simulink model "projeto_final"  (Simulink 6.3)
settings: Solver=ode3  StartTime=0  StopTime=5e-3  FixedStep=1e-7  RelTol=1e-3
undefined symbols (not defined in the file or in its folder): Fs, get
libraries: dsparch4 x1, commsynccomp2 x1, dspsnks4 x1
settings Model: LastModifiedBy=marco

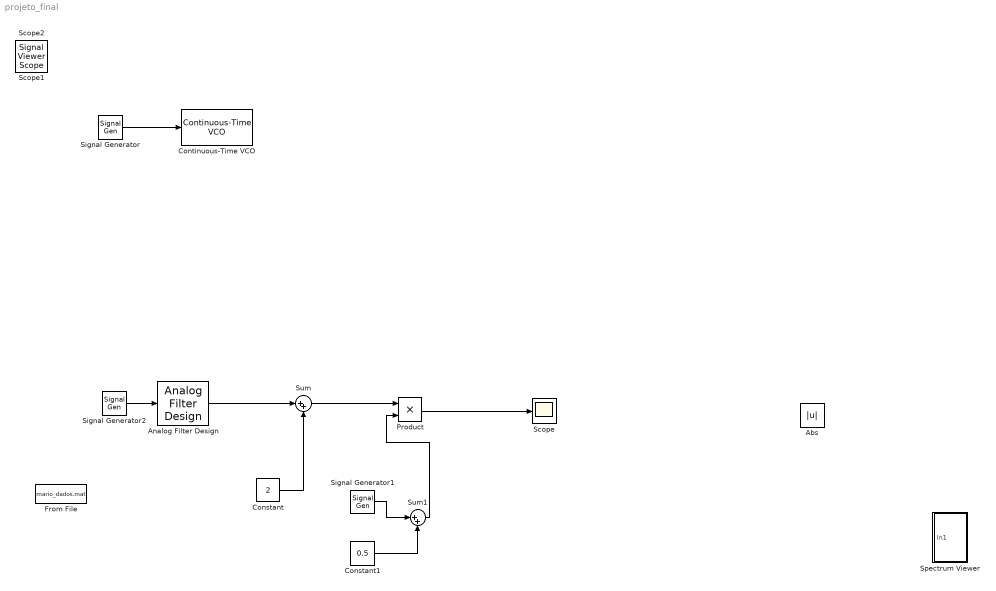
== system projeto_final ==
  Abs : Abs
  Analog Filter Design : dsparch4/Analog Filter Design  method=Butterworth  filttype=Lowpass  N=10  Wlo=2*pi*5e3  Whi=80  Rp=2  Rs=40
  Constant : Constant  Value=2
  Constant1 : Constant  Value=0.5
  Continuous-Time VCO : commsynccomp2/Continuous-Time VCO  Ac=1  Fc=1e5  Kc=40e3  Ph=0
  From File : FromFile  FileName=mario_dados.mat  SampleTime=0
  Product : Product  RndMeth=Zero
  Scope : Scope
  Signal Generator : SignalGenerator  WaveForm=square  Frequency=1e3
  Signal Generator1 : SignalGenerator  WaveForm=square  Amplitude=0.5  Frequency=1e5
  Signal Generator2 : SignalGenerator  Frequency=1e3
  "Spectrum Viewer " : Subsystem
  Sum : Sum  Inputs=|++
  Sum1 : Sum  Inputs=|++
  Scope1 : SignalViewerScope  IOType=viewer  RefreshTime=0.035000
  Scope2 : SignalViewerScope  IOType=viewer  RefreshTime=0.035000
  wires:
  Signal Generator/1 -> Continuous-Time VCO/1
  Analog Filter Design/1 -> Sum/1
  Constant/1 -> Sum/2
  Sum/1 -> Product/1
  Signal Generator1/1 -> Sum1/1
  Constant1/1 -> Sum1/2
  Sum1/1 -> Product/2
  Product/1 -> Scope/1
  Signal Generator2/1 -> Analog Filter Design/1

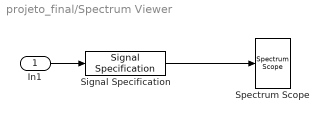
== system projeto_final/Spectrum Viewer  ==
  In1 : Inport
  Signal Specification : SignalSpecification  SampleTime=1e-7
  Spectrum Scope : dspsnks4/Spectrum Scope  DialogController=dspdialog.SpectrumScope  DialogControllerArgs=DataTag0  ScopeProperties=on  Domain=Frequency  HorizSpan=1  UseBuffer=on  BufferSize=1024  Overlap=64  inpFftLenInherit=off  FFTlength=128  numAvg=200  DisplayProperties=off  AxisGrid=on  Memory=off  FrameNumber=on  AxisLegend=off  AxisZoom=off  OpenScopeAtSimStart=on  OpenScopeImmediately=off  FigPos=get(0,'defaultfigureposition')  AxisProperties=off  XUnits=Hertz  XRange=[-Fs/2...Fs/2]  InheritXIncr=on  XIncr=1.0  XLabel=Samples  YUnits=dB  YLabel=Magnitude-squared, dB  LineProperties=off  wintypeSpecScope=Hann  RsSpecScope=50  betaSpecScope=5  winsampSpecScope=Periodic
      settings: YMin=-152.32674781566  YMax=20.0792208914918
  wires:
  In1/1 -> Signal Specification/1
  Signal Specification/1 -> Spectrum Scope/1
